simulink model "q910"  (Simulink 8.1)
settings: Solver=ode45  StartTime=0.0  StopTime=20  RelTol=1e-3
values from neighbouring files (symbols this model uses):
  a0 = 1    [task2.m]
  a1 = a10+delta_a1    (= 3.4)    [task2.m]
  a2 = a20+delta_a2    (= 4)    [task2.m]
  Ki = 1.5    [task2.m]
  Kq910 = K0+deltaK    (= 0.5)    [task2.m]
libraries: simulink x1
settings Model: Creator=Nelson  LastModifiedBy=Nelson
settings DataIOCC: SignalLoggingSaveFormat=Dataset
settings OptimizationCC: ExpressionDepthLimit=128
settings DebuggingCC: FcnCallInpInsideContextMsg=EnableAllAsError
settings GRTTargetCC: CombineOutputUpdateFcns=on  GRTInterface=off

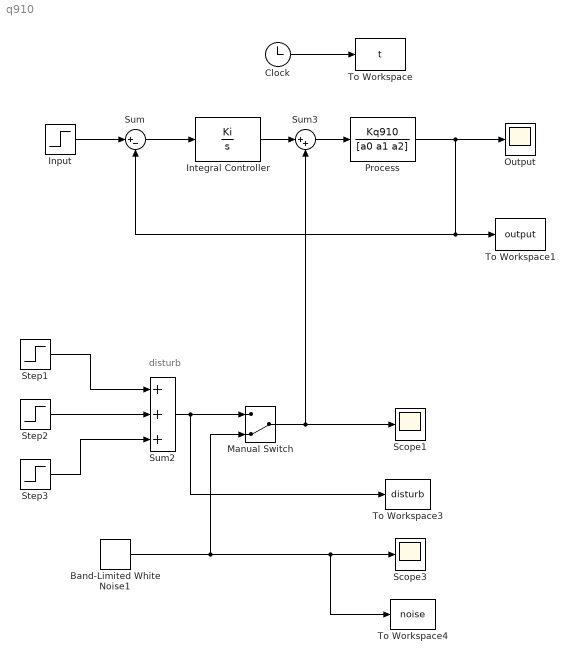
== system q910 ==
  note: disturb
  Band-Limited White Noise1 : simulink/Sources/Band-Limited White Noise  Cov=[0.01]  Ts=0.01  seed=[23341]
  Clock : Clock
  "Input " : Step  Time=0  SampleTime=0
  Integral Controller : TransferFcn  Numerator=Ki  Denominator=[1 0]
  Manual Switch : ManualSwitch  CurrentSetting=0
  "Output " : Scope
      settings: SaveName=outputScope  MaxDataPoints=500000
  Process : TransferFcn  Numerator=Kq910  Denominator=[a0 a1 a2]
  Scope1 : Scope
      settings: SaveName=ScopeData2
  Scope3 : Scope
      settings: SaveName=ScopeData3
  Step1 : Step  Time=0  After=-1  SampleTime=0
  Step2 : Step  Time=6  After=3  SampleTime=0
  Step3 : Step  Time=15  After=-1  SampleTime=0
  Sum : Sum  Inputs=|+-
  Sum2 : Sum  Inputs=+++
  Sum3 : Sum  Inputs=|++
  To Workspace : ToWorkspace  VariableName=t  SampleTime=-1
  To Workspace1 : ToWorkspace  VariableName=output  SampleTime=-1
  To Workspace3 : ToWorkspace  VariableName=disturb  SampleTime=-1
  To Workspace4 : ToWorkspace  VariableName=noise  SampleTime=-1
  wires:
  "Input "/1 -> Sum/1
  Process/1 -> "Output "/1, Sum/2, To Workspace1/1
  Sum/1 -> Integral Controller/1
  Clock/1 -> To Workspace/1
  Step2/1 -> Sum2/2
  Step1/1 -> Sum2/1
  Step3/1 -> Sum2/3
  Sum2/1 -> Manual Switch/1, To Workspace3/1
  Manual Switch/1 -> Scope1/1, Sum3/2
  Band-Limited White Noise1/1 -> Manual Switch/2, Scope3/1, To Workspace4/1
  Integral Controller/1 -> Sum3/1
  Sum3/1 -> Process/1
